simulink model "MultipleN_HotCase"  (R2018b)
settings: Solver=VariableStepAuto  StartTime=0.0  StopTime=time  RelTol=1e-3  EnableMultiTasking=on
values from neighbouring files (symbols this model uses):
  A_side = 2 * A_front    (= 0.02)    [MultipleNodes.m]    (also in OneNode.m)
  eps_1 = 0.81    [MultipleNodes.m]
  Qa_e1 = WS_e *A_side *alpha_1*a_e*REF    (= 7.23872468174)    [MultipleNodes.m]
  Qa_e2 = WS_e *A_side *alpha_2*a_e*REF    (= 7.23872468174)    [MultipleNodes.m]
  Qdiss_hot1 = 1.5    [MultipleNodes.m]
  Qdiss_hot2 = 0.2    [MultipleNodes.m]
  Qir_e1 = Wir_e*A_side *eps_1*REF    (= 3.6288)    [MultipleNodes.m]
  Qir_e2 = Wir_e*A_side *eps_2*REF    (= 3.6288)    [MultipleNodes.m]
  QS_e1 = WS_e *A_side * REF    (= 27.7345773247)    [MultipleNodes.m]
  QS_e2 = WS_e *A_side * REF    (= 27.7345773247)    [MultipleNodes.m]
  sigma = 5.67e-8    (= 5.67e-08)    [MultipleNodes.m]    (also in OneNode.m)
  T0 = mean(Ym)    [MultipleNodes.m]    (also in OneNode.m)
  T1_h = Y(2,2)    [MultipleNodes.m]
  T2_h = Y(1,2)    [MultipleNodes.m]
  Tds = 4    [MultipleNodes.m]    (also in OneNode.m)
libraries: fl_lib x39, nesl_utility x15
settings Model: Creator=Mauro  LastModifiedBy=aloisia
settings OptimizationCC: LifeSpan=inf
settings DebuggingCC: SFUnexpectedBacktrackingDiag=warning  SFNoUnconditionalDefaultTransitionDiag=warning
settings SFSimCC: SimUseLocalCustomCode=off
settings RTWCC: RTWUseLocalCustomCode=off
settings CodeAppCC: StateflowObjectComments=on
settings GRTTargetCC: TargetLangStandard=C89/C90 (ANSI)  GeneratePreprocessorConditionals=Disable all
settings ConfigComp: CovMetricSettings=dw  CovHtmlReporting=on  CovSaveCumulativeToWorkspaceVar=on  CovSaveSingleToWorkspaceVar=on  CovExternalEMLEnable=off
settings SimscapeCC: SimscapeNormalizeSystem=off

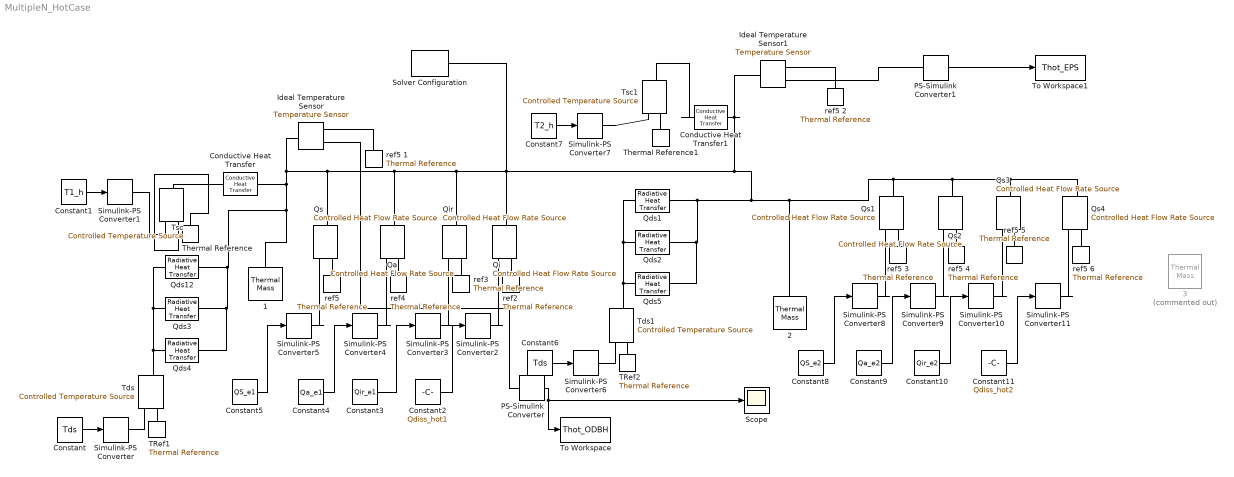
== system MultipleN_HotCase ==
  1 : fl_lib/Thermal/Thermal Elements/Thermal Mass  mass=M1 kg  sp_heat=447 J/kg/K  T_specify=on  T_priority=High  T=T0 K  T_nominal_specify=off  T_nominal_unit=K  T_nominal_value=1  Q_specify=off  Q_priority=None  Q=0 J/s  Q_nominal_specify=off  Q_nominal_unit=W  Q_nominal_value=1
  2 : fl_lib/Thermal/Thermal Elements/Thermal Mass  mass=M2 kg  sp_heat=447 J/kg/K  T_specify=on  T_priority=High  T=T0 K  T_nominal_specify=off  T_nominal_unit=K  T_nominal_value=1  Q_specify=off  Q_priority=None  Q=0 J/s  Q_nominal_specify=off  Q_nominal_unit=W  Q_nominal_value=1
  3 : fl_lib/Thermal/Thermal Elements/Thermal Mass  Commented=on  mass=M2 kg  sp_heat=447 J/kg/K  T_specify=on  T_priority=High  T=T0 K  T_nominal_specify=off  T_nominal_unit=K  T_nominal_value=1  Q_specify=off  Q_priority=None  Q=0 J/s  Q_nominal_specify=off  Q_nominal_unit=W  Q_nominal_value=1
  Conductive Heat Transfer : fl_lib/Thermal/Thermal Elements/Conductive Heat Transfer  area=0.01 m^2  thickness=0.01 m  th_cond=Gsc1 W/(m*K)  T_specify=off  T_priority=None  T=0 K  T_nominal_specify=off  T_nominal_unit=K  T_nominal_value=1  Q_specify=off  Q_priority=None  Q=0 J/s  Q_nominal_specify=off  Q_nominal_unit=W  Q_nominal_value=1
      settings: SourceProductName=Simscape
  Conductive Heat Transfer1 : fl_lib/Thermal/Thermal Elements/Conductive Heat Transfer  area=0.01 m^2  thickness=0.01 m  th_cond=Gsc2 W/(m*K)  T_specify=off  T_priority=None  T=0 K  T_nominal_specify=off  T_nominal_unit=K  T_nominal_value=1  Q_specify=off  Q_priority=None  Q=0 J/s  Q_nominal_specify=off  Q_nominal_unit=W  Q_nominal_value=1
      settings: SourceProductName=Simscape
  Constant : Constant  Value=Tds
  Constant1 : Constant  Value=T1_h
  Constant10 : Constant  Value=Qir_e2
  Constant11 : Constant  Value=Qdiss_hot2
  Constant2 : Constant  Value=Qdiss_hot1
  Constant3 : Constant  Value=Qir_e1
  Constant4 : Constant  Value=Qa_e1
  Constant5 : Constant  Value=QS_e1
  Constant6 : Constant  Value=Tds
  Constant7 : Constant  Value=T2_h
  Constant8 : Constant  Value=QS_e2
  Constant9 : Constant  Value=Qa_e2
  Ideal Temperature Sensor : fl_lib/Thermal/Thermal Sensors/Temperature Sensor
  Ideal Temperature Sensor1 : fl_lib/Thermal/Thermal Sensors/Temperature Sensor
  PS-Simulink Converter : nesl_utility/PS-Simulink Converter  PhysicalDomain=network_engine_domain  SubClassName=ps_output  LeftPortType=input  RightPortType=output  PseudoPeriodic=off  Frequencies=[]  Unit=1  AffineConversion=off
  PS-Simulink Converter1 : nesl_utility/PS-Simulink Converter  PhysicalDomain=network_engine_domain  SubClassName=ps_output  LeftPortType=input  RightPortType=output  PseudoPeriodic=off  Frequencies=[]  Unit=1  AffineConversion=off
  Qa : fl_lib/Thermal/Thermal Sources/Controlled Heat Flow Rate Source
      settings: SourceProductName=Simscape
  Qds1 : fl_lib/Thermal/Thermal Elements/Radiative Heat Transfer  area=2*A_side m^2  rad_tr_coeff=sigma*eps_1 W/(m^2*K^4)  T_specify=off  T_priority=None  T=0 K  T_nominal_specify=off  T_nominal_unit=K  T_nominal_value=1  Q_specify=off  Q_priority=None  Q=0 J/s  Q_nominal_specify=off  Q_nominal_unit=W  Q_nominal_value=1
      settings: SourceProductName=Simscape  SourceProductBaseCode=SS
  Qds12 : fl_lib/Thermal/Thermal Elements/Radiative Heat Transfer  area=2*A_side m^2  rad_tr_coeff=sigma*eps_1 W/(m^2*K^4)  T_specify=off  T_priority=None  T=0 K  T_nominal_specify=off  T_nominal_unit=K  T_nominal_value=1  Q_specify=off  Q_priority=None  Q=0 J/s  Q_nominal_specify=off  Q_nominal_unit=W  Q_nominal_value=1
      settings: SourceProductName=Simscape  SourceProductBaseCode=SS
  Qds{2..5} (4 alike) : fl_lib/Thermal/Thermal Elements/Radiative Heat Transfer  area=A_front m^2  rad_tr_coeff=sigma*eps_1 W/(m^2*K^4)  T_specify=off  T_priority=None  T=0 K  T_nominal_specify=off  T_nominal_unit=K  T_nominal_value=1  Q_specify=off  Q_priority=None  Q=0 J/s  Q_nominal_specify=off  Q_nominal_unit=W  Q_nominal_value=1
      settings: SourceProductName=Simscape  SourceProductBaseCode=SS
  Qi : fl_lib/Thermal/Thermal Sources/Controlled Heat Flow Rate Source
      settings: SourceProductName=Simscape
  Qir : fl_lib/Thermal/Thermal Sources/Controlled Heat Flow Rate Source
      settings: SourceProductName=Simscape
  Qs{,1..4} (5 alike) : fl_lib/Thermal/Thermal Sources/Controlled Heat Flow Rate Source
      settings: SourceProductName=Simscape
  Scope : Scope
  Simulink-PS Converter{,1..11} (12 alike) : nesl_utility/Simulink-PS Converter  PhysicalDomain=network_engine_domain  SubClassName=ps_input  LeftPortType=input  RightPortType=output  PseudoPeriodic=off  Frequencies=[]  NoiseDistribution=none  NoiseParameters=[]  Unit=1  AffineConversion=off  FilteringAndDerivatives=zero  SimscapeFilterOrder=1  InputFilterTimeConstant=0.001  UdotUserProvided=1
  Solver Configuration : nesl_utility/Solver Configuration  PhysicalDomain=network_engine_domain  SubClassName=solver  LeftPortType=input  RightPortType=generic  Tones=[]  Harmonics=[]  SimulateNoise=off  Profile=off  UseLocalSampling=off  EnableSwitchedLinearOptims=on  FrequencyDomain=off  UseCCode=off  RelTol=0.001  AbsTol=1e-06  MinStep=1e-09  ToWorkspace=off  RevertToSquareIcSolve=off  NumHomotopyIterations=100  PhasorMode=off  PhasorModeNumHarmonics=1  DoDC=off  ResidualTolerance=1e-09  UseLocalSolver=off  LocalSolverChoice=NE_BACKWARD_EULER_ADVANCER  LocalSolverSampleTime=0.001  DoFixedCost=off  MaxNonlinIter=3  MaxModeIter=2  LinearAlgebra=Sparse  EquationFormulation=NE_TIME_EF  DelaysMemoryBudget=1024  AutomaticFiltering=on  FilteringTimeConstant=0.001  PartitionStorageMethod=AS_NEEDED  PartitionMemoryBudget=1024
  TRef1 : fl_lib/Thermal/Thermal Elements/Thermal Reference
  TRef2 : fl_lib/Thermal/Thermal Elements/Thermal Reference
  Tds : fl_lib/Thermal/Thermal Sources/Controlled Temperature Source
      settings: SourceProductName=Simscape
  Tds1 : fl_lib/Thermal/Thermal Sources/Controlled Temperature Source
      settings: SourceProductName=Simscape
  Thermal Reference : fl_lib/Thermal/Thermal Elements/Thermal Reference
  Thermal Reference1 : fl_lib/Thermal/Thermal Elements/Thermal Reference
  To Workspace : ToWorkspace  VariableName=Thot_ODBH  SaveFormat=Timeseries  SampleTime=-1
  To Workspace1 : ToWorkspace  VariableName=Thot_EPS  SaveFormat=Timeseries  SampleTime=-1
  Tsc : fl_lib/Thermal/Thermal Sources/Controlled Temperature Source
      settings: SourceProductName=Simscape
  Tsc1 : fl_lib/Thermal/Thermal Sources/Controlled Temperature Source
      settings: SourceProductName=Simscape
  ref2 : fl_lib/Thermal/Thermal Elements/Thermal Reference
  "ref3 " : fl_lib/Thermal/Thermal Elements/Thermal Reference
  ref4 : fl_lib/Thermal/Thermal Elements/Thermal Reference
  ref5 {,1..6} (7 alike) : fl_lib/Thermal/Thermal Elements/Thermal Reference
  wires:
  Constant/1 -> Simulink-PS Converter/1
  Constant1/1 -> Simulink-PS Converter1/1
  Constant2/1 -> Simulink-PS Converter2/1
  Constant3/1 -> Simulink-PS Converter3/1
  Constant4/1 -> Simulink-PS Converter4/1
  Constant5/1 -> Simulink-PS Converter5/1
  PS-Simulink Converter/1 -> To Workspace/1, Scope/1
  Constant7/1 -> Simulink-PS Converter7/1
  Constant6/1 -> Simulink-PS Converter6/1
  PS-Simulink Converter1/1 -> To Workspace1/1
  Constant8/1 -> Simulink-PS Converter8/1
  Constant9/1 -> Simulink-PS Converter9/1
  Constant10/1 -> Simulink-PS Converter10/1
  Constant11/1 -> Simulink-PS Converter11/1
  connections:
  Thermal Reference/LConn1 -- Tsc/RConn2
  TRef1/LConn1 -- Tds/RConn2
  Simulink-PS Converter/RConn1 -- Tds/RConn1
  Simulink-PS Converter1/RConn1 -- Tsc/RConn1
  Conductive Heat Transfer/LConn1 -- Tsc/LConn1
  ref2/LConn1 -- Qi/RConn2
  Simulink-PS Converter2/RConn1 -- Qi/RConn1
  Simulink-PS Converter3/RConn1 -- Qir/RConn1
  "ref3 "/LConn1 -- Qir/RConn2
  ref4/LConn1 -- Qa/RConn2
  Simulink-PS Converter4/RConn1 -- Qa/RConn1
  Simulink-PS Converter5/RConn1 -- Qs/RConn1
  "ref5 "/LConn1 -- Qs/RConn2
  Qds12/LConn1 -- Qds3/LConn1 -- Qds4/LConn1 -- Tds/LConn1
  ref5 1/LConn1 -- Ideal Temperature Sensor/RConn1
  Ideal Temperature Sensor/RConn2 -- PS-Simulink Converter/LConn1
  Tds1/LConn1 -- Qds5/LConn1 -- Qds1/LConn1 -- Qds2/LConn1
  Conductive Heat Transfer1/RConn1 -- Ideal Temperature Sensor1/LConn1 -- Qs2/LConn1 -- Qs3/LConn1 -- Qs4/LConn1 -- Qs1/LConn1 -- 2/LConn1 -- Qds5/RConn1 -- Qds2/RConn1 -- Qds1/RConn1 -- Conductive Heat Transfer/RConn1 -- 1/LConn1 -- Qds4/RConn1 -- Qds3/RConn1 -- Qds12/RConn1 -- Ideal Temperature Sensor/LConn1 -- Qs/LConn1 -- Qa/LConn1 -- Qir/LConn1 -- Solver Configuration/RConn1 -- Qi/LConn1
  TRef2/LConn1 -- Tds1/RConn2
  Simulink-PS Converter6/RConn1 -- Tds1/RConn1
  Simulink-PS Converter7/RConn1 -- Tsc1/RConn1
  Thermal Reference1/LConn1 -- Tsc1/RConn2
  ref5 2/LConn1 -- Ideal Temperature Sensor1/RConn1
  PS-Simulink Converter1/LConn1 -- Ideal Temperature Sensor1/RConn2
  Conductive Heat Transfer1/LConn1 -- Tsc1/LConn1
  Simulink-PS Converter8/RConn1 -- Qs1/RConn1
  ref5 3/LConn1 -- Qs1/RConn2
  Simulink-PS Converter9/RConn1 -- Qs2/RConn1
  ref5 4/LConn1 -- Qs2/RConn2
  Simulink-PS Converter10/RConn1 -- Qs3/RConn1
  ref5 5/LConn1 -- Qs3/RConn2
  Simulink-PS Converter11/RConn1 -- Qs4/RConn1
  ref5 6/LConn1 -- Qs4/RConn2
